simulink model "SLEW1"  (Simulink 3.00)
settings: Solver=ode45  SolverMode=SingleTasking  StartTime=0.0  StopTime=40  MaxStep=.010  RelTol=1e-3  AbsTol=1e-3
undefined symbols (not defined in the file or in its folder): slew
settings Model: TimeSaveName=t  SaveOutput=off

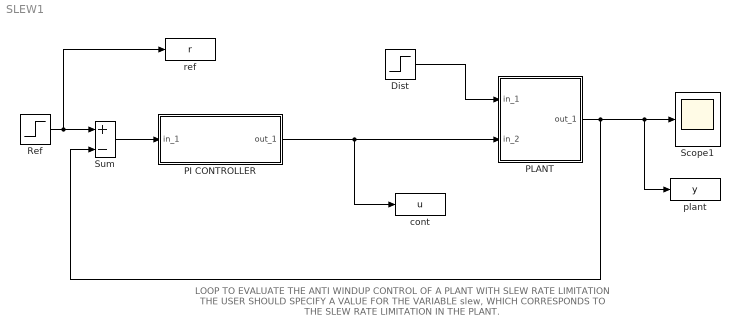
== system SLEW1 ==
  note: LOOP TO EVALUATE THE ANTI WINDUP CONTROL OF A PLANT WITH SLEW RATE LIMITATION
      | THE USER SHOULD SPECIFY A VALUE FOR THE VARIABLE slew, WHICH CORRESPONDS TO THE SLEW RATE
      | LIMITATION IN THE PLANT.
  Dist : Step  Time=20  Before=0  After=1  SampleTime=0
  PI CONTROLLER : Subsystem  mask(PI controller){@1=0.5, @2=1.5, @3=slew}
      mask prompts: @1 "Prop gain Kp:"; @2 "Integral time Tr:"; @3 "slew rate limit s_max:"
      mask help: PI controller
      mask init:
      | Kp=@1;Tr=@2;slewc=@3;
      mask Help: PI controller with anti wind up feature for slew rate limitation
      mask Display: disp('PI+A.WU ')
  PLANT : Subsystem
      mask Type: PLANT
      mask Display: disp('Plant')
  Ref : Step  Time=1  Before=0  After=1  SampleTime=0
  Scope1 : Scope
      settings: TickLabels=on  TimeRange=40.000000  YMin=-2  YMax=2  SaveToWorkspace=off  SaveName=ScopeData  DataFormat=Matrix
  Sum : Sum  Inputs=+-  SaturateOnIntegerOverflow=on
  cont : ToWorkspace  VariableName=u  SampleTime=0  SaveFormat=Matrix
      settings: Buffer=10000
  plant : ToWorkspace  VariableName=y  SampleTime=0  SaveFormat=Matrix
      settings: Buffer=6000
  ref : ToWorkspace  VariableName=r  SampleTime=0  SaveFormat=Matrix
      settings: Buffer=10000
  wires:
  Sum/1 -> PI CONTROLLER/1(in_1)
  Dist/1 -> PLANT/1(in_1)
  PI CONTROLLER/1(out_1) -> PLANT/2(in_2), cont/1
  Ref/1 -> Sum/1, ref/1
  PLANT/1(out_1) -> Scope1/1, plant/1, Sum/2

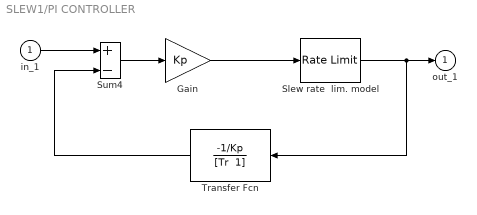
== system SLEW1/PI CONTROLLER ==
  in_1 : Inport  Port=1  PortWidth=-1  SampleTime=-1  DataType=auto
      settings: SignalType=auto
  Gain : Gain  Gain=Kp  SaturateOnIntegerOverflow=on
  Slew rate  lim. model : RateLimiter  RisingSlewLimit=slewc  FallingSlewLimit=-slewc
  Sum4 : Sum  Inputs=+-  SaturateOnIntegerOverflow=on
  Transfer Fcn : TransferFcn  Orientation=left  Numerator=-1/Kp  Denominator="[Tr  1]"
  out_1 : Outport  Port=1  InitialOutput=0
  wires:
  Transfer Fcn/1 -> Sum4/2
  Gain/1 -> Slew rate  lim. model/1
  Sum4/1 -> Gain/1
  in_1/1 -> Sum4/1
  Slew rate  lim. model/1 -> out_1/1, Transfer Fcn/1

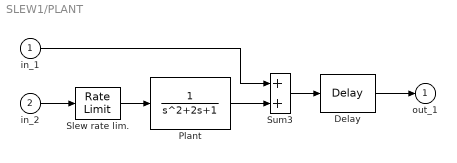
== system SLEW1/PLANT ==
  in_1 : Inport  Port=1  PortWidth=-1  SampleTime=-1  DataType=auto
      settings: SignalType=auto
  in_2 : Inport  Port=2  PortWidth=-1  SampleTime=-1  DataType=auto
      settings: SignalType=auto
  Delay : TransportDelay  DelayTime=1.  InitialInput=0  BufferSize=4096
  Plant : TransferFcn  Numerator=1  Denominator="[1 2  1 ]"
  Slew rate lim. : RateLimiter  RisingSlewLimit=slew  FallingSlewLimit=-slew
  Sum3 : Sum  Inputs=++  SaturateOnIntegerOverflow=on
  out_1 : Outport  Port=1  InitialOutput=0
  wires:
  Plant/1 -> Sum3/2
  Sum3/1 -> Delay/1
  Slew rate lim./1 -> Plant/1
  in_1/1 -> Sum3/1
  Delay/1 -> out_1/1
  in_2/1 -> Slew rate lim./1
